simulink model "rsxSatSim"  (R2025b)
settings: Solver=FixedStepAuto  StartTime=0.0  StopTime=simIn.runTime  FixedStep=simIn.simTs  MaxStep=simIn.simTs*1.01  MinStep=simIn.simTs*0.99  RelTol=1e-3
undefined symbols (not defined in the file): simIn
libraries: simulink_extras x4, aerolibutil x2
settings Model: Creator=layer  LastModifiedBy=layer
settings SolverCC: InitialStep=simIn.simTs

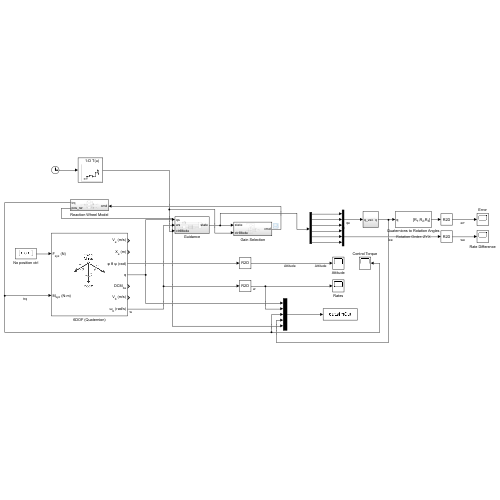
[thumbnail: Simulink's stored preview of the top-level diagram]
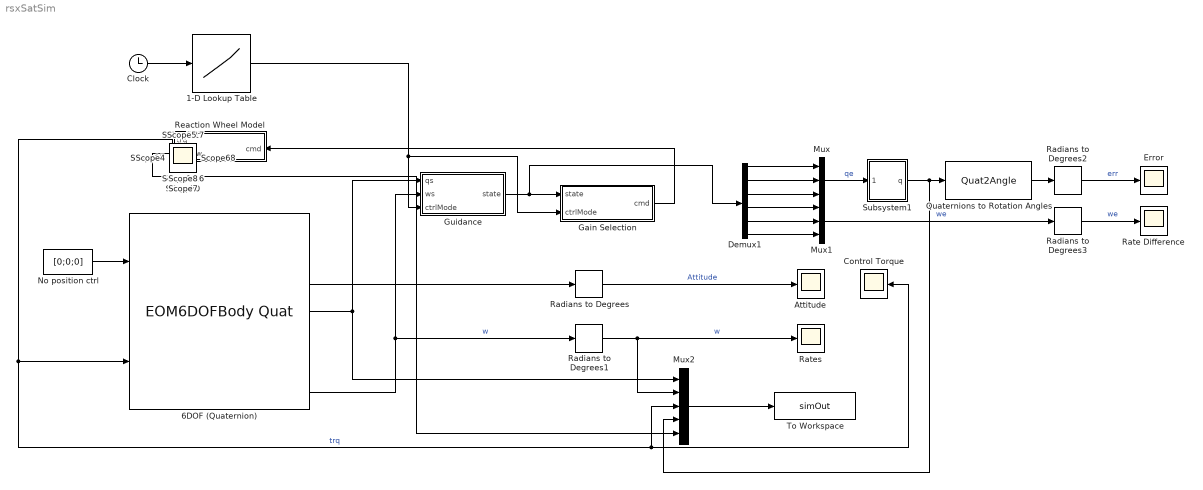
== system rsxSatSim ==
  1-D Lookup Table : Lookup_n-D  NumberOfTableDimensions=1  BreakpointsForDimension1=simIn.ctrlTimes  Table=simIn.ctrlModes  InterpMethod=Flat  InternalRulePriority=Speed  RndMeth=Simplest
  6DOF (Quaternion) : EOM6DOFBodyQuat  eul_0=simIn.att0  pm_0=simIn.w0  inertia=simIn.Jv
  Attitude : Scope
      settings: ActiveDisplayYMinimum=-224.99806520869984  ActiveDisplayYMaximum=224.99224421980961
  Clock : Clock
  Control Torque : Scope
      settings: ActiveDisplayYMinimum=-0.0021836250000000002  ActiveDisplayYMaximum=0.0021836250000000002
  Demux1 : Demux  Outputs=6
  Error : Scope
      settings: ActiveDisplayYMinimum=-224.44973384717642  ActiveDisplayYMaximum=224.92501685686642  DataLoggingVariableName=ScopeData10
  Gain Selection : Subsystem
  Guidance : Subsystem
  Mux : Mux  Inputs=3
  Mux1 : Mux  Inputs=3
  Mux2 : Mux  Inputs=5
  No position ctrl : Constant  Value=[0;0;0]  SampleTime=0.1
  Quaternions to Rotation Angles : Quat2Angle
      settings: AttributesFormatString=Rotation Order: %<rotationOrder>
  Radians to Degrees{,1..3} (4 alike) : simulink_extras/Transformations/Radians to Degrees
  Rate Difference : Scope
      settings: ActiveDisplayYMinimum=-40.910953183921549  ActiveDisplayYMaximum=68.200174417725734  DataLoggingVariableName=ScopeData11
  Rates : Scope
      settings: ActiveDisplayYMinimum=-64.026338777179  ActiveDisplayYMaximum=52.288247800897906  DataLoggingVariableName=ScopeData3
  Reaction Wheel Model : Subsystem
  Subsystem1 : Subsystem
  To Workspace : ToWorkspace  VariableName=simOut  SaveFormat=Structure With Time  SampleTime=-1
      settings: Decimation=4
  Scope{,1,4..8,11..20} (17 alike) : Scope
      Scope settings: ActiveDisplayYMinimum=0.75000000000000011  ActiveDisplayYMaximum=3.25  DataLoggingVariableName=ScopeData2
      Scope1 settings: ActiveDisplayYMinimum=-70.685834705805419  ActiveDisplayYMaximum=7.853981634290073  DataLoggingVariableName=ScopeData5
      Scope11 settings: ActiveDisplayYMinimum=-28.203339898062783  ActiveDisplayYMaximum=72.94687451289127  DataLoggingVariableName=ScopeData12
      Scope12 settings: ActiveDisplayYMinimum=-1  ActiveDisplayYMaximum=1  DataLoggingVariableName=ScopeData13
      Scope13 settings: ActiveDisplayYMinimum=0.62500000000000011  ActiveDisplayYMaximum=4.375  DataLoggingVariableName=ScopeData14
      Scope14 settings: ActiveDisplayYMinimum=-1  ActiveDisplayYMaximum=1  DataLoggingVariableName=ScopeData15
      Scope15 settings: ActiveDisplayYMinimum=0.9  ActiveDisplayYMaximum=1.1  DataLoggingVariableName=ScopeData16
      Scope16 settings: ActiveDisplayYMinimum=2.9999997550806867  ActiveDisplayYMaximum=3.0000005765285795  DataLoggingVariableName=ScopeData17
      Scope17 settings: ActiveDisplayYMinimum=-1  ActiveDisplayYMaximum=1  DataLoggingVariableName=ScopeData18
      Scope18 settings: ActiveDisplayYMinimum=-2696.549570576135  ActiveDisplayYMaximum=577.99919358818386  DataLoggingVariableName=ScopeData19
      Scope19 settings: ActiveDisplayYMinimum=-165.38821421047822  ActiveDisplayYMaximum=50.61993225668445  DataLoggingVariableName=ScopeData20
      Scope20 settings: ActiveDisplayYMinimum=-2676.8735438003177  ActiveDisplayYMaximum=407.80893853555068  DataLoggingVariableName=ScopeData21
      Scope4 settings: ActiveDisplayYMinimum=-8.7499999999999982  ActiveDisplayYMaximum=78.75  DataLoggingVariableName=ScopeData4
      Scope5 settings: ActiveDisplayYMinimum=-1  ActiveDisplayYMaximum=1  DataLoggingVariableName=ScopeData6
      Scope6 settings: ActiveDisplayYMinimum=-1  ActiveDisplayYMaximum=1  DataLoggingVariableName=ScopeData7
      Scope7 settings: ActiveDisplayYMinimum=62.82695846941229  ActiveDisplayYMaximum=62.927197592987632  DataLoggingVariableName=ScopeData8
      Scope8 settings: ActiveDisplayYMinimum=-1  ActiveDisplayYMaximum=1  DataLoggingVariableName=ScopeData9
  wires:
  No position ctrl/1 -> 6DOF (Quaternion)/1
  6DOF (Quaternion)/4 -> Guidance/1(qs), Mux2/1
  6DOF (Quaternion)/3 -> Radians to Degrees/1
  Radians to Degrees/1 -> Attitude/1  "Attitude"
  Radians to Degrees1/1 -> Rates/1, Mux2/2  "w"
  Mux2/1 -> To Workspace/1
  Reaction Wheel Model/1(trq) -> 6DOF (Quaternion)/2, Mux2/3, Control Torque/1  "trq"
  Gain Selection/1(cmd) -> Reaction Wheel Model/1(cmd)
  6DOF (Quaternion)/7 -> Radians to Degrees1/1, Guidance/2(ws)  "w"
  Clock/1 -> 1-D Lookup Table/1
  Demux1/5 -> Mux1/2
  Demux1/3 -> Mux/3
  Mux1/1 -> Radians to Degrees3/1  "we"
  Guidance/1(state) -> Demux1/1, Gain Selection/1(state)
  Demux1/2 -> Mux/2
  Demux1/4 -> Mux1/1
  Demux1/6 -> Mux1/3
  Demux1/1 -> Mux/1
  Quaternions to Rotation Angles/1 -> Radians to Degrees2/1
  Radians to Degrees2/1 -> Error/1  "err"
  Radians to Degrees3/1 -> Rate Difference/1  "we"
  1-D Lookup Table/1 -> Guidance/3(ctrlMode), Gain Selection/2(ctrlMode)
  Mux/1 -> Subsystem1/1(q_vec)  "qe"
  Subsystem1/1(q) -> Mux2/4, Quaternions to Rotation Angles/1
  Reaction Wheel Model/2(pos_rw) -> Mux2/5

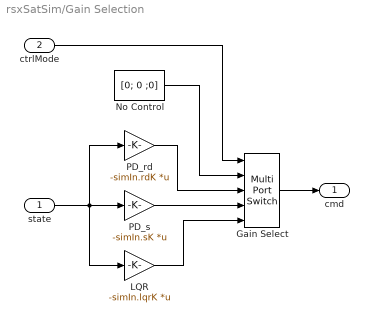
== system rsxSatSim/Gain Selection ==
  state : Inport
  ctrlMode : Inport  Port=2
  Gain Select : MultiPortSwitch  DataPortOrder=Zero-based contiguous  Inputs=4  zeroidx=on  SaturateOnIntegerOverflow=off  InputSameDT=off
  LQR : Gain  Gain=-simIn.lqrK  Multiplication=Matrix(K*u)
  No Control : Constant  Value=[0; 0 ;0]
  PD_rd : Gain  Gain=-simIn.rdK  Multiplication=Matrix(K*u)
  PD_s : Gain  Gain=-simIn.sK  Multiplication=Matrix(K*u)
  cmd : Outport
  wires:
  state/1 -> LQR/1, PD_s/1, PD_rd/1
  PD_s/1 -> Gain Select/4
  LQR/1 -> Gain Select/5
  Gain Select/1 -> cmd/1
  PD_rd/1 -> Gain Select/3
  No Control/1 -> Gain Select/2
  ctrlMode/1 -> Gain Select/1

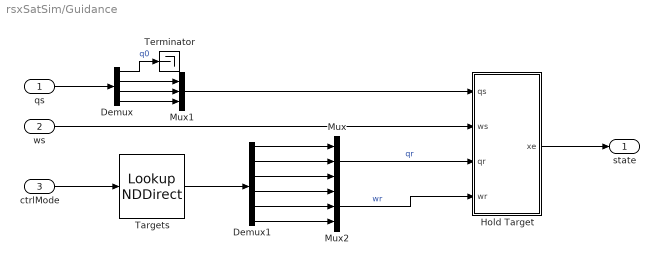
== system rsxSatSim/Guidance ==
  qs : Inport
  ws : Inport  Port=2
  ctrlMode : Inport  Port=3
  Demux : Demux
  Demux1 : Demux  Outputs=6
  Hold Target : Subsystem
  Mux : Mux  Inputs=3
  Mux1 : Mux  Inputs=3
  Mux2 : Mux  Inputs=3
  Targets : LookupNDDirect  InputsSelectThisObjectFromTable=Vector  Table=simIn.trgt'
  Terminator : Terminator
  state : Outport
  wires:
  Mux1/1 -> Hold Target/1(qs)
  Hold Target/1(xe) -> state/1
  ws/1 -> Hold Target/2(ws)
  qs/1 -> Demux/1
  Demux/2 -> Mux1/1
  Demux/3 -> Mux1/2
  Demux/4 -> Mux1/3
  Demux/1 -> Terminator/1  "q0"
  Mux/1 -> Hold Target/3(qr)  "qr"
  Demux1/2 -> Mux/2
  Demux1/4 -> Mux2/1
  Demux1/5 -> Mux2/2
  Demux1/3 -> Mux/3
  Demux1/6 -> Mux2/3
  Mux2/1 -> Hold Target/4(wr)  "wr"
  Targets/1 -> Demux1/1
  Demux1/1 -> Mux/1
  ctrlMode/1 -> Targets/1

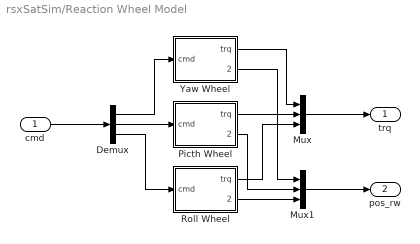
== system rsxSatSim/Reaction Wheel Model ==
  cmd : Inport
  Demux : Demux  Outputs=3
  Mux : Mux  Inputs=3
  Mux1 : Mux  Inputs=3
  Picth Wheel : Subsystem
  Roll Wheel : Subsystem
  Yaw Wheel : Subsystem
  trq : Outport
  pos_rw : Outport  Port=2
  wires:
  Demux/1 -> Yaw Wheel/1(cmd)
  Demux/2 -> Picth Wheel/1(cmd)
  Demux/3 -> Roll Wheel/1(cmd)
  Picth Wheel/1(trq) -> Mux/2
  Yaw Wheel/1(trq) -> Mux/1
  Roll Wheel/1(trq) -> Mux/3
  Mux/1 -> trq/1
  cmd/1 -> Demux/1
  Roll Wheel/2(pos_rw) -> Mux1/3
  Picth Wheel/2(pos_rw) -> Mux1/2
  Yaw Wheel/2(pos_rw) -> Mux1/1
  Mux1/1 -> pos_rw/1

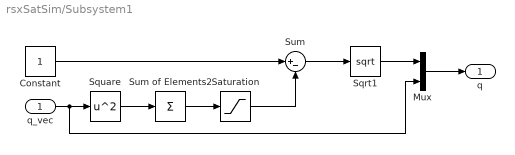
== system rsxSatSim/Subsystem1 ==
  q_vec : Inport
  Constant : Constant
  Mux : Mux  Inputs=2
  Saturation : Saturate  UpperLimit=1  LowerLimit=0
  Sqrt1 : Sqrt
  Square : Math  Operator=square
  Sum : Sum  Inputs=|+-
  Sum of Elements2 : Sum  Inputs=+
  q : Outport
  wires:
  q_vec/1 -> Mux/2, Square/1
  Sum/1 -> Sqrt1/1
  Constant/1 -> Sum/1
  Sum of Elements2/1 -> Saturation/1
  Square/1 -> Sum of Elements2/1
  Sqrt1/1 -> Mux/1
  Saturation/1 -> Sum/2
  Mux/1 -> q/1

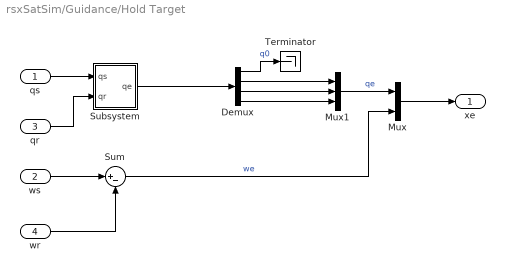
== system rsxSatSim/Guidance/Hold Target ==
  qs : Inport
  ws : Inport  Port=2
  qr : Inport  Port=3
  wr : Inport  Port=4
  Demux : Demux
  Mux : Mux  Inputs=2
  Mux1 : Mux  Inputs=3
  Subsystem : Subsystem
  Sum : Sum  Inputs=|+-
  Terminator : Terminator
  xe : Outport
  wires:
  Mux1/1 -> Mux/1  "qe"
  Demux/4 -> Mux1/3
  Demux/2 -> Mux1/1
  Demux/1 -> Terminator/1  "q0"
  Demux/3 -> Mux1/2
  Mux/1 -> xe/1
  qs/1 -> Subsystem/1(qs)
  Subsystem/1(qe) -> Demux/1
  qr/1 -> Subsystem/2(qr)
  ws/1 -> Sum/1
  wr/1 -> Sum/2
  Sum/1 -> Mux/2  "we"

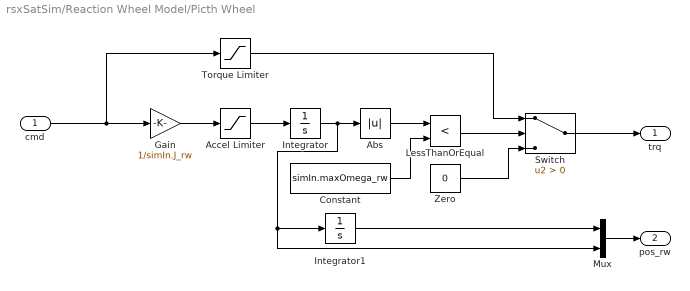
== system rsxSatSim/Reaction Wheel Model/Picth Wheel ==
  cmd : Inport
  Abs : Abs  SaturateOnIntegerOverflow=off
  Accel Limiter : Saturate  UpperLimit=simIn.alpha_rw  LowerLimit=-simIn.alpha_rw
  Constant : Constant  Value=simIn.maxOmega_rw
  Gain : Gain  Gain=1/simIn.J_rw
  Integrator : Integrator  LimitOutput=on  UpperSaturationLimit=simIn.maxOmega_rw  LowerSaturationLimit=-simIn.maxOmega_rw
  Integrator1 : Integrator
  LessThanOrEqual : RelationalOperator  Operator=<  OutDataTypeStr=boolean  RndMeth=Simplest  InputSameDT=off
  Mux : Mux  Inputs=2
  Switch : Switch  Criteria=u2 > Threshold  SaturateOnIntegerOverflow=off  InputSameDT=off
  Torque Limiter : Saturate  UpperLimit=simIn.trq_rw  LowerLimit=-simIn.trq_rw
  Zero : Constant  Value=0  OutDataTypeStr=Inherit: Inherit via back propagation
  trq : Outport
  pos_rw : Outport  Port=2
  wires:
  cmd/1 -> Torque Limiter/1, Gain/1
  Gain/1 -> Accel Limiter/1
  Torque Limiter/1 -> Switch/1
  Constant/1 -> LessThanOrEqual/2
  Zero/1 -> Switch/3
  LessThanOrEqual/1 -> Switch/2
  Accel Limiter/1 -> Integrator/1
  Switch/1 -> trq/1
  Abs/1 -> LessThanOrEqual/1
  Mux/1 -> pos_rw/1
  Integrator1/1 -> Mux/1
  Integrator/1 -> Mux/2, Integrator1/1, Abs/1

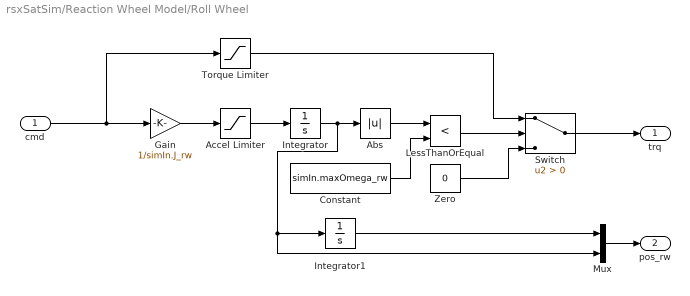
== system rsxSatSim/Reaction Wheel Model/Roll Wheel ==
  cmd : Inport
  Abs : Abs  SaturateOnIntegerOverflow=off
  Accel Limiter : Saturate  UpperLimit=simIn.alpha_rw  LowerLimit=-simIn.alpha_rw
  Constant : Constant  Value=simIn.maxOmega_rw
  Gain : Gain  Gain=1/simIn.J_rw
  Integrator : Integrator  LimitOutput=on  UpperSaturationLimit=simIn.maxOmega_rw  LowerSaturationLimit=-simIn.maxOmega_rw
  Integrator1 : Integrator
  LessThanOrEqual : RelationalOperator  Operator=<  OutDataTypeStr=boolean  RndMeth=Simplest  InputSameDT=off
  Mux : Mux  Inputs=2
  Switch : Switch  Criteria=u2 > Threshold  SaturateOnIntegerOverflow=off  InputSameDT=off
  Torque Limiter : Saturate  UpperLimit=simIn.trq_rw  LowerLimit=-simIn.trq_rw
  Zero : Constant  Value=0  OutDataTypeStr=Inherit: Inherit via back propagation
  trq : Outport
  pos_rw : Outport  Port=2
  wires:
  cmd/1 -> Torque Limiter/1, Gain/1
  Gain/1 -> Accel Limiter/1
  Torque Limiter/1 -> Switch/1
  Constant/1 -> LessThanOrEqual/2
  Zero/1 -> Switch/3
  LessThanOrEqual/1 -> Switch/2
  Accel Limiter/1 -> Integrator/1
  Switch/1 -> trq/1
  Abs/1 -> LessThanOrEqual/1
  Mux/1 -> pos_rw/1
  Integrator1/1 -> Mux/1
  Integrator/1 -> Mux/2, Integrator1/1, Abs/1

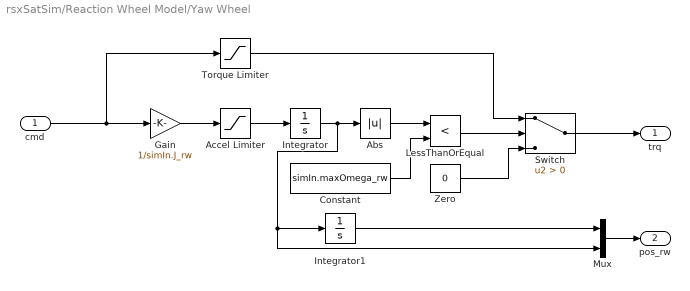
== system rsxSatSim/Reaction Wheel Model/Yaw Wheel ==
  cmd : Inport
  Abs : Abs  SaturateOnIntegerOverflow=off
  Accel Limiter : Saturate  UpperLimit=simIn.alpha_rw  LowerLimit=-simIn.alpha_rw
  Constant : Constant  Value=simIn.maxOmega_rw
  Gain : Gain  Gain=1/simIn.J_rw
  Integrator : Integrator  LimitOutput=on  UpperSaturationLimit=simIn.maxOmega_rw  LowerSaturationLimit=-simIn.maxOmega_rw
  Integrator1 : Integrator
  LessThanOrEqual : RelationalOperator  Operator=<  OutDataTypeStr=boolean  RndMeth=Simplest  InputSameDT=off
  Mux : Mux  Inputs=2
  Switch : Switch  Criteria=u2 > Threshold  SaturateOnIntegerOverflow=off  InputSameDT=off
  Torque Limiter : Saturate  UpperLimit=simIn.trq_rw  LowerLimit=-simIn.trq_rw
  Zero : Constant  Value=0  OutDataTypeStr=Inherit: Inherit via back propagation
  trq : Outport
  pos_rw : Outport  Port=2
  wires:
  cmd/1 -> Torque Limiter/1, Gain/1
  Gain/1 -> Accel Limiter/1
  Integrator/1 -> Mux/2, Integrator1/1, Abs/1
  Constant/1 -> LessThanOrEqual/2
  Zero/1 -> Switch/3
  LessThanOrEqual/1 -> Switch/2
  Accel Limiter/1 -> Integrator/1
  Switch/1 -> trq/1
  Abs/1 -> LessThanOrEqual/1
  Integrator1/1 -> Mux/1
  Torque Limiter/1 -> Switch/1
  Mux/1 -> pos_rw/1

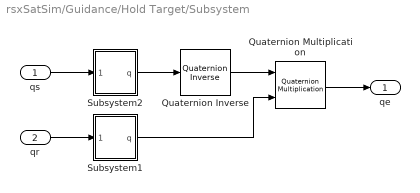
== system rsxSatSim/Guidance/Hold Target/Subsystem ==
  qs : Inport
  qr : Inport  Port=2
  Quaternion Inverse : aerolibutil/Quaternion Inverse
  Quaternion Multiplication : aerolibutil/Quaternion Multiplication
  Subsystem1 : Subsystem
  Subsystem2 : Subsystem
  qe : Outport
  wires:
  Quaternion Inverse/1 -> Quaternion Multiplication/1
  qr/1 -> Subsystem1/1(q_vec)
  qs/1 -> Subsystem2/1(q_vec)
  Quaternion Multiplication/1 -> qe/1
  Subsystem2/1(q) -> Quaternion Inverse/1
  Subsystem1/1(q) -> Quaternion Multiplication/2

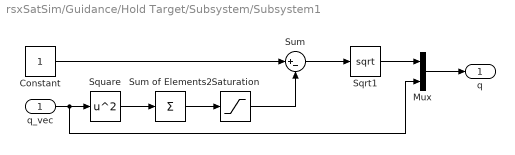
== system rsxSatSim/Guidance/Hold Target/Subsystem/Subsystem1 ==
  q_vec : Inport
  Constant : Constant
  Mux : Mux  Inputs=2
  Saturation : Saturate  UpperLimit=1  LowerLimit=0
  Sqrt1 : Sqrt
  Square : Math  Operator=square
  Sum : Sum  Inputs=|+-
  Sum of Elements2 : Sum  Inputs=+
  q : Outport
  wires:
  q_vec/1 -> Mux/2, Square/1
  Sum/1 -> Sqrt1/1
  Constant/1 -> Sum/1
  Sum of Elements2/1 -> Saturation/1
  Square/1 -> Sum of Elements2/1
  Sqrt1/1 -> Mux/1
  Saturation/1 -> Sum/2
  Mux/1 -> q/1

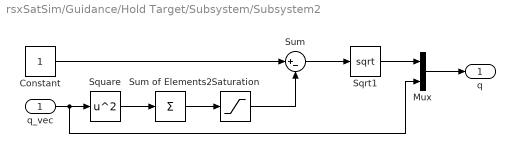
== system rsxSatSim/Guidance/Hold Target/Subsystem/Subsystem2 ==
  q_vec : Inport
  Constant : Constant
  Mux : Mux  Inputs=2
  Saturation : Saturate  UpperLimit=1  LowerLimit=0
  Sqrt1 : Sqrt
  Square : Math  Operator=square
  Sum : Sum  Inputs=|+-
  Sum of Elements2 : Sum  Inputs=+
  q : Outport
  wires:
  q_vec/1 -> Mux/2, Square/1
  Sum/1 -> Sqrt1/1
  Constant/1 -> Sum/1
  Sum of Elements2/1 -> Saturation/1
  Square/1 -> Sum of Elements2/1
  Sqrt1/1 -> Mux/1
  Saturation/1 -> Sum/2
  Mux/1 -> q/1
